simulink model "TrafficLightMDB"  (R2018b)
settings: Solver=FixedStepDiscrete  StartTime=0.0  StopTime=inf  RelTol=1e-3
settings Model: Creator=dahroug  LastModifiedBy=dahroug
settings OptimizationCC: DefaultParameterBehavior=Inlined  EnhancedBackFolding=on  PassReuseOutputArgsAs=Individual arguments  OptimizeBlockOrder=speed  DifferentSizesBufferReuse=on  OptimizationCustomize=off
settings DebuggingCC: UnderspecifiedInitializationDetection=Classic  MergeDetectMultiDrivingBlocksExec=none  ParameterTunabilityLossMsg=error
settings ModelReferenceCC: PropagateSignalLabelsOutOfModel=off
settings SFSimCC: MATLABDynamicMemAlloc=off
settings RTWCC: SystemTargetFile=ert.tlc  GenCodeOnly=on  TemplateMakefile=ert_default_tmf  GenerateReport=on  IncludeHyperlinkInReport=on  LaunchReport=on  GenerateTraceInfo=on  GenerateTraceReport=on  GenerateTraceReportSl=on  GenerateTraceReportSf=on  GenerateTraceReportEml=on
settings CodeAppCC: ForceParamTrailComments=on  IgnoreCustomStorageClasses=off  OperatorAnnotations=on  SimulinkDataObjDesc=on  SFDataObjDesc=on  InsertBlockDesc=on
settings ERTTargetCC: TargetLangStandard=C99 (ISO)  GenerateSampleERTMain=on  InlinedParameterPlacement=NonHierarchical  ERTCustomFileTemplate=example_file_process.tlc

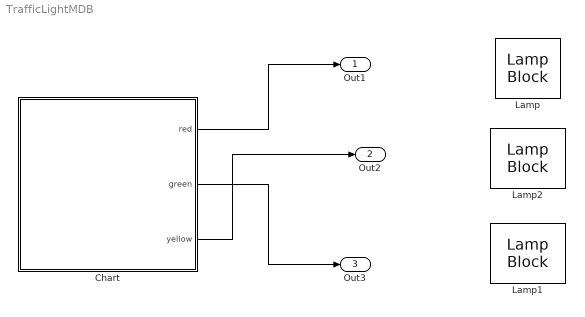
== system TrafficLightMDB ==
  Chart : Stateflow chart  TreatAsAtomicUnit=on
  Lamp : LampBlock  WebBlockId=2
  Lamp1 : LampBlock  WebBlockId=3
  Lamp2 : LampBlock  WebBlockId=4
  Out1 : Outport  OutDataTypeStr=uint8
  Out2 : Outport  Port=2  OutDataTypeStr=uint8
  Out3 : Outport  Port=3  OutDataTypeStr=uint8
  wires:
  Chart/1(red) -> Out1/1
  Chart/2(green) -> Out3/1
  Chart/3(yellow) -> Out2/1

== stateflow chart TrafficLightMDB/Chart ==
  state stop
    du:
    red = (1);
    green = (0);
    yellow = (0);
    ex:
    red = (0);
    green = (0);
    yellow = (0)
  state start
    du:
    red = (0);
    green = (1);
    yellow = (0);
    ex:
    red = (0);
    green = (0);
    yellow = (0)
  state ready
    du:
    red = (0);
    green = (0);
    yellow = (1);
    ex:
    red = (0);
    green = (0);
    yellow = (0)
  start -> stop : after(3000,msec)
  (default) -> stop
  ready -> start : after(3000,msec)
  stop -> ready : after(3000,msec)
  data: red output uint8; green output uint8; yellow output uint8
